simulink model "model1"  (R2022a)
settings: Solver=VariableStepAuto  StartTime=0.0  StopTime=10.0  RelTol=1e-3
values from neighbouring files (symbols this model uses):
  A = [-a_1  1 ... (first row only)    [config.m]
  A_0 = [-k_1 1 ... (first row only)    [config.m]
  b = [b_1 ... (first row only)    [config.m]
  C = [1 0]    [config.m]
  gamma = 10    [config.m]    (also in task.m = 0.02)
  Ks = [1, k_1, k_0]    [config.m]
  theta = [k_0-a_0, k_1-a_1, b_0, b_1]    [config.m]
  x_0 = [0 ... (first row only)    [config.m]
settings Model: LastModifiedBy=Vvlad
settings OptimizationCC: BlockReduction=off  BooleanDataType=off
settings DebuggingCC: SaveWithParameterizedLinksMsg=none  UnderspecifiedInitializationDetection=Classic  MergeDetectMultiDrivingBlocksExec=none  SignalResolutionControl=TryResolveAllWithWarning  UnconnectedInputMsg=warning  UnconnectedOutputMsg=warning  UnconnectedLineMsg=warning
settings HardwareCC: TargetUnknown=on
settings ModelReferenceCC: PropagateSignalLabelsOutOfModel=off
settings RTWCC: DLArmComputeVersion=19.05

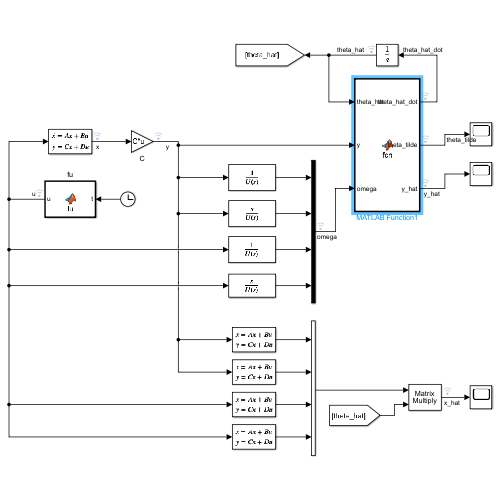
[thumbnail: Simulink's stored preview of the top-level diagram]
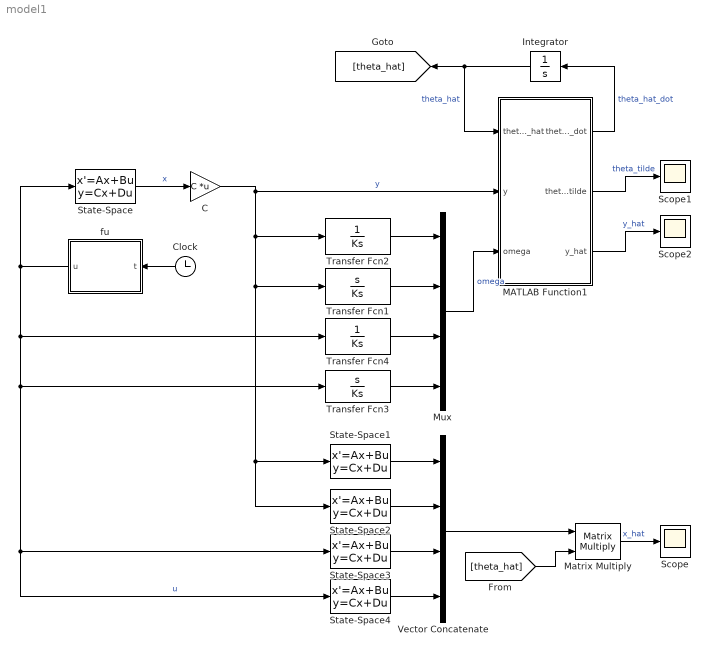
== system model1 ==
  C : Gain  Gain=C  Multiplication=Matrix(K*u)
  Clock : Clock
  Integrator : Integrator  InitialCondition=[0;0;0;0]
  MATLAB Function1 : MATLAB Function  TreatAsAtomicUnit=on
  Matrix Multiply : Product  Multiplication=Matrix(*)
  Mux : Mux
  Scope : Scope
  Scope1 : Scope
  Scope2 : Scope
  State-Space : StateSpace  A=A  B=b  C=eye(2)  D=[0;0]  InitialCondition=x_0
  State-Space1 : StateSpace  A=A_0  B=[0;1]  C=eye(2)  D=[0; 0]  InitialCondition=0
  State-Space2 : StateSpace  A=A_0  B=[1;0]  C=eye(2)  D=[0; 0]  InitialCondition=0
  State-Space3 : StateSpace  A=A_0  B=[0;1]  C=eye(2)  D=[0; 0]  InitialCondition=0
  State-Space4 : StateSpace  A=A_0  B=[1;0]  C=eye(2)  D=[0; 0]  InitialCondition=0
  Transfer Fcn1 : TransferFcn  Numerator=[1 0]  Denominator=Ks
  Transfer Fcn2 : TransferFcn  Numerator=1  Denominator=Ks
  Transfer Fcn3 : TransferFcn  Numerator=[1 0]  Denominator=Ks
  Transfer Fcn4 : TransferFcn  Numerator=1  Denominator=Ks
  Vector Concatenate : Concatenate  NumInputs=4  Mode=Multidimensional array  ConcatenateDimension=2
  fu : MATLAB Function  TreatAsAtomicUnit=on
  wires:
  State-Space/1 -> C/1  "x"
  MATLAB Function1/1(theta_hat_dot) -> Integrator/1  "theta_hat_dot"
  Integrator/1 -> MATLAB Function1/1(theta_hat), [theta_hat]  "theta_hat"
  Clock/1 -> fu/1(t)
  fu/1(u) -> State-Space/1, Transfer Fcn4/1, State-Space4/1, State-Space3/1, Transfer Fcn3/1  "u"
  C/1 -> Transfer Fcn2/1, State-Space2/1, State-Space1/1, Transfer Fcn1/1, MATLAB Function1/2(y)  "y"
  Transfer Fcn2/1 -> Mux/1
  Mux/1 -> MATLAB Function1/3(omega)  "omega"
  Transfer Fcn1/1 -> Mux/2
  Transfer Fcn4/1 -> Mux/3
  Transfer Fcn3/1 -> Mux/4
  MATLAB Function1/3(y_hat) -> Scope2/1  "y_hat"
  State-Space1/1 -> Vector Concatenate/1
  State-Space2/1 -> Vector Concatenate/2
  State-Space3/1 -> Vector Concatenate/3
  State-Space4/1 -> Vector Concatenate/4
  Matrix Multiply/1 -> Scope/1  "x_hat"
  [theta_hat] -> Matrix Multiply/2
  Vector Concatenate/1 -> Matrix Multiply/1
  MATLAB Function1/2(theta_tilde) -> Scope1/1  "theta_tilde"

== matlab function model1/MATLAB Function1 ==
  data: theta_hat input; theta_hat_dot output; theta_tilde output; y input; omega input; y_hat output; gamma parameter; theta parameter
function [theta_hat_dot, theta_tilde, y_hat]  = fcn(theta_hat, y, omega, gamma, theta)

y_hat = theta_hat'*omega;
epsilon = y - y_hat;
theta_hat_dot = gamma*omega*epsilon;
theta_tilde = theta - theta_hat;

== matlab function model1/fu ==
  data: t input; u output
function u = fu(t)
u = sin(t)+0.5*cos(2*t);
